simulink model "exponential"  (R2024b)
settings: Solver=VariableStepAuto  StartTime=0.0  StopTime=10.0  RelTol=1e-3
settings Model: Creator=shohei  LastModifiedBy=shohei

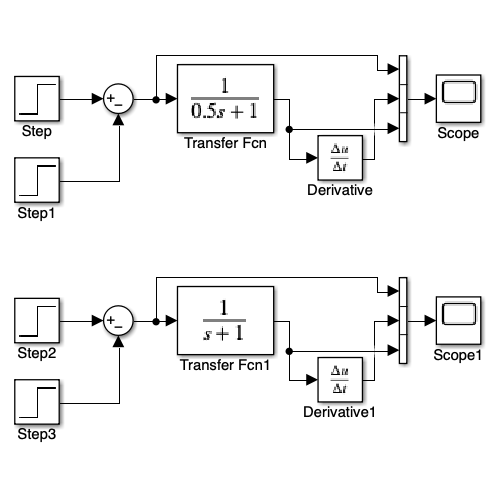
[thumbnail: Simulink's stored preview of the top-level diagram]
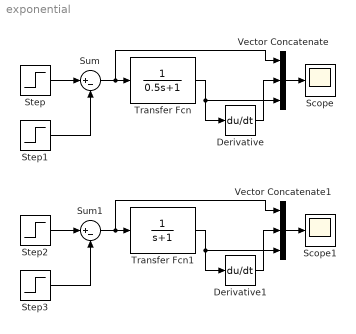
== system exponential ==
  Derivative : Derivative
  Derivative1 : Derivative
  Scope : Scope
  Scope1 : Scope
  Step : Step  SampleTime=0
  Step1 : Step  Time=5  SampleTime=0
  Step2 : Step  SampleTime=0
  Step3 : Step  Time=5  SampleTime=0
  Sum : Sum  Inputs=|+-
  Sum1 : Sum  Inputs=|+-
  Transfer Fcn : TransferFcn  Denominator=[0.5 1]
  Transfer Fcn1 : TransferFcn  Denominator=[1 1]
  Vector Concatenate : Concatenate  NumInputs=3
  Vector Concatenate1 : Concatenate  NumInputs=3
  wires:
  Step/1 -> Sum/1
  Step1/1 -> Sum/2
  Sum/1 -> Vector Concatenate/1, Transfer Fcn/1
  Transfer Fcn/1 -> Vector Concatenate/3, Derivative/1
  Derivative/1 -> Vector Concatenate/2
  Vector Concatenate/1 -> Scope/1
  Sum1/1 -> Vector Concatenate1/1, Transfer Fcn1/1
  Step3/1 -> Sum1/2
  Transfer Fcn1/1 -> Vector Concatenate1/3, Derivative1/1
  Step2/1 -> Sum1/1
  Derivative1/1 -> Vector Concatenate1/2
  Vector Concatenate1/1 -> Scope1/1
